simulink library "SurfLib"  (R2016b)
settings: Solver=ode45  StartTime=0.0  StopTime=10.0  RelTol=1e-3  EnableMultiTasking=on
undefined symbols (not defined in the file or in its folder): surf
undefined symbols (not defined in the file): AC
libraries: Surf_Lib x4, simulink x1
settings Model: Creator=austinmurch  LastModifiedBy=rega0051
settings DataIOCC: LimitDataPoints=on  SaveFormat=Array  SignalLoggingSaveFormat=ModelDataLogs
settings OptimizationCC: ExpressionDepthLimit=2147483647  LifeSpan=inf  SimCompilerOptimization=on
settings DebuggingCC: UnderspecifiedInitializationDetection=Classic  MergeDetectMultiDrivingBlocksExec=none  SolverPrmCheckMsg=warning  FcnCallInpInsideContextMsg=warning  StateNameClashWarn=warning  StrictBusMsg=Warning  SFUnexpectedBacktrackingDiag=warning  SFNoUnconditionalDefaultTransitionDiag=warning  SFExecutionAtInitializationDiag=none
settings HardwareCC: ProdBitPerPointer=32  ProdBitPerSizeT=32  ProdBitPerPtrDiffT=32  ProdLargestAtomicFloat=None  ProdIntDivRoundTo=Undefined  ProdEndianess=Unspecified  ProdWordSize=32  ProdHWDeviceType=32-bit Generic
settings ModelReferenceCC: PropagateSignalLabelsOutOfModel=off
settings GRTTargetCC: TargetLangStandard=C89/C90 (ANSI)  GeneratePreprocessorConditionals=Disable all  CombineOutputUpdateFcns=off  GRTInterface=on
settings ConfigComp: CovMetricSettings=dw  CovHtmlReporting=on  CovSaveCumulativeToWorkspaceVar=on  CovSaveSingleToWorkspaceVar=on  CovExternalEMLEnable=off

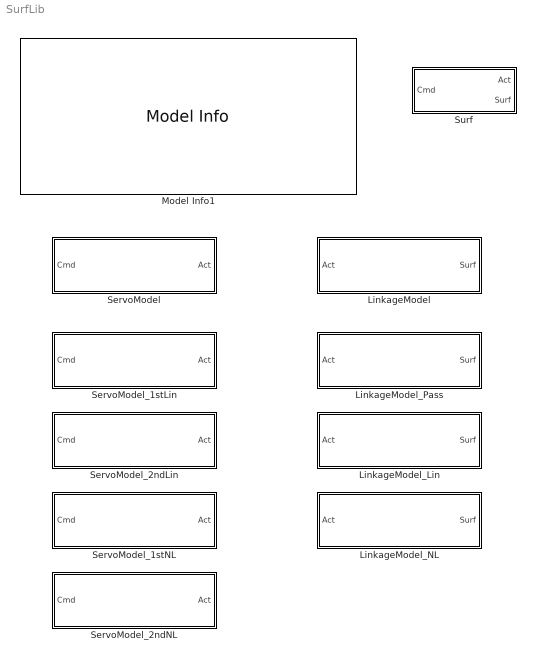
== system SurfLib ==
  LinkageModel : Subsystem  BlockChoice=LinkageModel_Lin
      settings: TemplateBlock=self  MemberBlocks=LinkageModel_Lin,LinkageModel_NL,LinkageModel_Pass
  LinkageModel_Lin : Subsystem  VariantControl=VarLink_Lin
  LinkageModel_NL : Subsystem  VariantControl=VarLink_Lin
  LinkageModel_Pass : Subsystem  VariantControl=AC_TYPE_SIMPLE
  Model Info1 : simulink/Model-Wide Utilities/Model Info  Frame=on  DisplayStringWithTags=|  HorizontalTextAlignment=Left  LeftAlignmentValue=0.02  SourceBlockDiagram=Surf_Lib  TagMaxNumber=20
      | MODEL INFORMATION
      | Control Surface Model Library
      | 
      | University of Minnesota
      | Aerospace Engineering and Mechanics
      | Copyright 2017 Regents of the University of Minnesota. All rights reserved.
      | 
      | == Info ==
      | Last modified by %<LastModifiedBy> on %<LastModificationDate>
  ServoModel : Subsystem  BlockChoice=ServoModel_1stLin
      settings: TemplateBlock=self  MemberBlocks=ServoModel_1stLin,ServoModel_1stNL,ServoModel_2ndLin,ServoModel_2ndNL
  ServoModel_1stLin : Subsystem  VariantControl=AC_TYPE_SIMPLE
  ServoModel_1stNL : Subsystem  VariantControl=VarServo_NL1
  ServoModel_2ndLin : Subsystem  VariantControl=VarServo_NL1
  ServoModel_2ndNL : Subsystem  VariantControl=VarServo_NL1
  Surf : Subsystem  mask{surf=AC.Surf.ailL}
      mask prompts: surf "Surface Structure:"

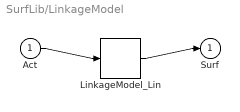
== system SurfLib/LinkageModel ==
  Act : Inport
  LinkageModel_Lin : Surf_Lib/LinkageModel_Lin  VariantControl=VarLink_Lin
  Surf : Outport
  wires:
  Act/1 -> LinkageModel_Lin/1
  LinkageModel_Lin/1 -> Surf/1

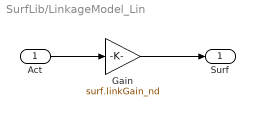
== system SurfLib/LinkageModel_Lin ==
  Act : Inport
  Gain : Gain  Gain=surf.linkGain_nd
      settings: AttributesFormatString=%<Gain>
  Surf : Outport  PortDimensions=1
  wires:
  Act/1 -> Gain/1
  Gain/1 -> Surf/1

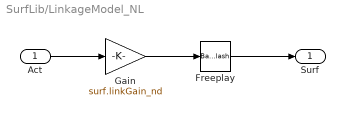
== system SurfLib/LinkageModel_NL ==
  Act : Inport
  Freeplay : Backlash  BacklashWidth=surf.linkFreeplay_rad  InitialOutput=surf.init_rad
      settings: AttributesFormatString=|
      | %<BacklashWidth>
      | %<InitialOutput>
  Gain : Gain  Gain=surf.linkGain_nd
      settings: AttributesFormatString=%<Gain>
  Surf : Outport  PortDimensions=1
  wires:
  Gain/1 -> Freeplay/1
  Act/1 -> Gain/1
  Freeplay/1 -> Surf/1

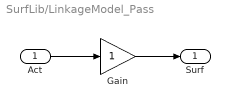
== system SurfLib/LinkageModel_Pass ==
  Act : Inport
  Gain : Gain
      settings: AttributesFormatString=%<Gain>
  Surf : Outport  PortDimensions=1
  wires:
  Act/1 -> Gain/1
  Gain/1 -> Surf/1

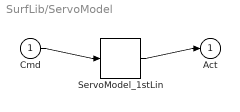
== system SurfLib/ServoModel ==
  Cmd : Inport
  ServoModel_1stLin : Surf_Lib/ServoModel_1stLin  VariantControl=AC_TYPE_SIMPLE
  Act : Outport
  wires:
  Cmd/1 -> ServoModel_1stLin/1
  ServoModel_1stLin/1 -> Act/1

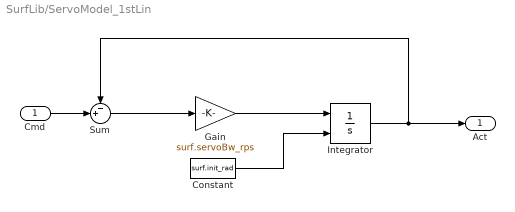
== system SurfLib/ServoModel_1stLin ==
  Cmd : Inport
  Constant : Constant  Value=surf.init_rad
      settings: AttributesFormatString=%<Value>
  Gain : Gain  Gain=surf.servoBw_rps  SaturateOnIntegerOverflow=on  OutDataTypeStr=Inherit: Same as input  ParamDataTypeStr=Inherit: Same as input
      settings: AttributesFormatString=%<Gain>
  Integrator : Integrator  InitialConditionSource=external  InitialCondition=surf.init_rad  UpperSaturationLimit=Inf  LowerSaturationLimit=-Inf  IgnoreLimit=on  ContinuousStateAttributes='servoPosition'
      settings: AttributesFormatString=State: %<ContinuousStateAttributes>
  Sum : Sum  Inputs=-+|  SaturateOnIntegerOverflow=on  InputSameDT=on  OutDataTypeStr=Inherit: Same as first input
  Act : Outport  PortDimensions=1
  wires:
  Gain/1 -> Integrator/1
  Sum/1 -> Gain/1
  Integrator/1 -> Sum/1, Act/1
  Cmd/1 -> Sum/2
  Constant/1 -> Integrator/2

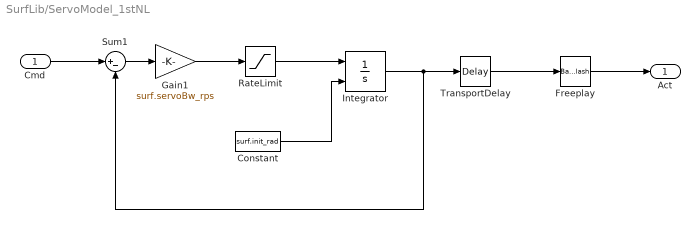
== system SurfLib/ServoModel_1stNL ==
  Cmd : Inport
  Constant : Constant  Value=surf.init_rad
      settings: AttributesFormatString=%<Value>
  Freeplay : Backlash  BacklashWidth=surf.servoFreeplay_rad  InitialOutput=surf.init_rad
      settings: AttributesFormatString=|
      | %<BacklashWidth>
      | %<InitialOutput>
  Gain1 : Gain  Gain=surf.servoBw_rps  SaturateOnIntegerOverflow=on  OutDataTypeStr=Inherit: Same as input  ParamDataTypeStr=Inherit: Same as input
      settings: AttributesFormatString=%<Gain>
  Integrator : Integrator  InitialConditionSource=external  InitialCondition=surf.init_rad  LimitOutput=on  UpperSaturationLimit=surf.servoLimPos_rad  LowerSaturationLimit=surf.servoLimNeg_rad  IgnoreLimit=on
  RateLimit : Saturate  UpperLimit=surf.servoRateLim_rps  LowerLimit=-surf.servoRateLim_rps
      settings: AttributesFormatString=|
      | %<LowerLimit>
      | %<UpperLimit>
  Sum1 : Sum  Inputs=|+-  SaturateOnIntegerOverflow=on  InputSameDT=on  OutDataTypeStr=Inherit: Same as first input
  TransportDelay : TransportDelay  DelayTime=surf.servoTimeDelay_s  InitialOutput=surf.init_rad  TransDelayFeedthrough=on  PadeOrder=2
      settings: AttributesFormatString=|
      | %<DelayTime>
      | %<InitialOutput>
  Act : Outport  PortDimensions=1
  wires:
  Gain1/1 -> RateLimit/1
  Sum1/1 -> Gain1/1
  Integrator/1 -> Sum1/2, TransportDelay/1
  Cmd/1 -> Sum1/1
  Constant/1 -> Integrator/2
  RateLimit/1 -> Integrator/1
  Freeplay/1 -> Act/1
  TransportDelay/1 -> Freeplay/1

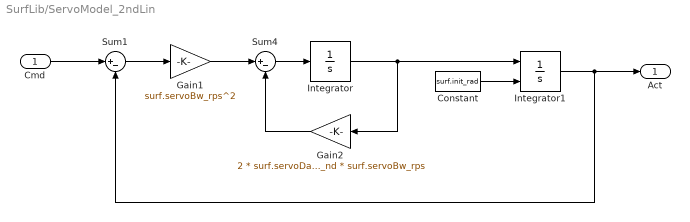
== system SurfLib/ServoModel_2ndLin ==
  Cmd : Inport
  Constant : Constant  Value=surf.init_rad
      settings: AttributesFormatString=%<Value>
  Gain1 : Gain  Gain=surf.servoBw_rps^2  SaturateOnIntegerOverflow=on  OutDataTypeStr=Inherit: Same as input  ParamDataTypeStr=Inherit: Same as input
      settings: AttributesFormatString=%<Gain>
  Gain2 : Gain  Gain=2 * surf.servoDamp_nd * surf.servoBw_rps  SaturateOnIntegerOverflow=on  OutDataTypeStr=Inherit: Same as input  ParamDataTypeStr=Inherit: Same as input
      settings: AttributesFormatString=%<Gain>
  Integrator : Integrator  UpperSaturationLimit=surf.servoRateLim_rps  LowerSaturationLimit=-surf.servoRateLim_rps  IgnoreLimit=on
  Integrator1 : Integrator  InitialConditionSource=external  InitialCondition=surf.init_rad  UpperSaturationLimit=surf.servoLimPos_rad  LowerSaturationLimit=surf.servoLimNeg_rad  IgnoreLimit=on
  Sum1 : Sum  Inputs=|+-  SaturateOnIntegerOverflow=on  InputSameDT=on  OutDataTypeStr=Inherit: Same as first input
  Sum4 : Sum  Inputs=|+-  SaturateOnIntegerOverflow=on  InputSameDT=on  OutDataTypeStr=Inherit: Same as first input
  Act : Outport  PortDimensions=1
  wires:
  Sum1/1 -> Gain1/1
  Cmd/1 -> Sum1/1
  Constant/1 -> Integrator1/2
  Gain1/1 -> Sum4/1
  Integrator1/1 -> Act/1, Sum1/2
  Integrator/1 -> Gain2/1, Integrator1/1
  Sum4/1 -> Integrator/1
  Gain2/1 -> Sum4/2

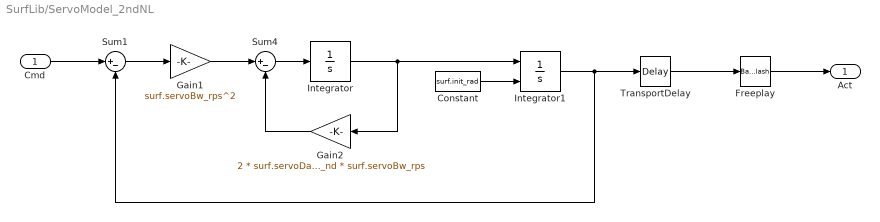
== system SurfLib/ServoModel_2ndNL ==
  Cmd : Inport
  Constant : Constant  Value=surf.init_rad
      settings: AttributesFormatString=%<Value>
  Freeplay : Backlash  BacklashWidth=surf.servoFreeplay_rad  InitialOutput=surf.init_rad
      settings: AttributesFormatString=|
      | %<BacklashWidth>
      | %<InitialOutput>
  Gain1 : Gain  Gain=surf.servoBw_rps^2  SaturateOnIntegerOverflow=on  OutDataTypeStr=Inherit: Same as input  ParamDataTypeStr=Inherit: Same as input
      settings: AttributesFormatString=%<Gain>
  Gain2 : Gain  Gain=2 * surf.servoDamp_nd * surf.servoBw_rps  SaturateOnIntegerOverflow=on  OutDataTypeStr=Inherit: Same as input  ParamDataTypeStr=Inherit: Same as input
      settings: AttributesFormatString=%<Gain>
  Integrator : Integrator  LimitOutput=on  UpperSaturationLimit=surf.servoRateLim_rps  LowerSaturationLimit=-surf.servoRateLim_rps  IgnoreLimit=on
  Integrator1 : Integrator  InitialConditionSource=external  InitialCondition=surf.init_rad  LimitOutput=on  UpperSaturationLimit=surf.servoLimPos_rad  LowerSaturationLimit=surf.servoLimNeg_rad  IgnoreLimit=on
  Sum1 : Sum  Inputs=|+-  SaturateOnIntegerOverflow=on  InputSameDT=on  OutDataTypeStr=Inherit: Same as first input
  Sum4 : Sum  Inputs=|+-  SaturateOnIntegerOverflow=on  InputSameDT=on  OutDataTypeStr=Inherit: Same as first input
  TransportDelay : TransportDelay  DelayTime=surf.servoTimeDelay_s  InitialOutput=surf.init_rad  TransDelayFeedthrough=on  PadeOrder=2
      settings: AttributesFormatString=|
      | %<DelayTime>
      | %<InitialOutput>
  Act : Outport  PortDimensions=1
  wires:
  Gain2/1 -> Sum4/2
  Sum4/1 -> Integrator/1
  Integrator/1 -> Integrator1/1, Gain2/1
  TransportDelay/1 -> Freeplay/1
  Freeplay/1 -> Act/1
  Gain1/1 -> Sum4/1
  Constant/1 -> Integrator1/2
  Cmd/1 -> Sum1/1
  Integrator1/1 -> TransportDelay/1, Sum1/2
  Sum1/1 -> Gain1/1

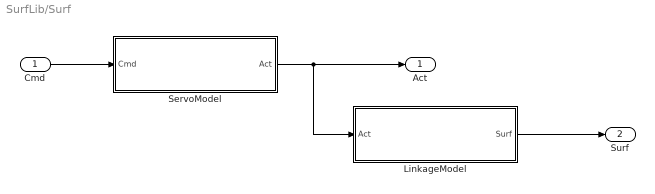
== system SurfLib/Surf ==
  Cmd : Inport
  LinkageModel : Subsystem  BlockChoice=LinkageModel_Lin
      settings: AttributesFormatString=%<BlockChoice>  TemplateBlock=Surf_Lib/LinkageModel  MemberBlocks=LinkageModel_Lin,LinkageModel_NL,LinkageModel_Pass
  ServoModel : Subsystem  BlockChoice=ServoModel_2ndLin
      settings: AttributesFormatString=%<BlockChoice>  TemplateBlock=Surf_Lib/ServoModel  MemberBlocks=ServoModel_1stLin,ServoModel_1stNL,ServoModel_2ndLin,ServoModel_2ndNL
  Act : Outport
  Surf : Outport  Port=2
  wires:
  Cmd/1 -> ServoModel/1(Cmd)
  ServoModel/1(Act) -> LinkageModel/1(Act), Act/1
  LinkageModel/1(Surf) -> Surf/1

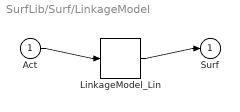
== system SurfLib/Surf/LinkageModel ==
  Act : Inport
  LinkageModel_Lin : Surf_Lib/LinkageModel_Lin  VariantControl=VarLink_Lin
  Surf : Outport
  wires:
  Act/1 -> LinkageModel_Lin/1
  LinkageModel_Lin/1 -> Surf/1

== system SurfLib/Surf/ServoModel ==
  Cmd : Inport
  ServoModel_2ndLin : Surf_Lib/ServoModel_2ndLin  VariantControl=VarServo_NL1
  Act : Outport
  wires:
  Cmd/1 -> ServoModel_2ndLin/1
  ServoModel_2ndLin/1 -> Act/1
